simulink model "Proper"  (R2018b)
settings: Solver=VariableStepAuto  StartTime=0.0  StopTime=20.0  RelTol=1e-3
values from neighbouring files (symbols this model uses):
  g = 9.81    [ABS.m]    (also in dane.m)
  Jw = 0.01    [ABS.m]    (also in dane.m)
  K = 1000    [ABS.m]
  mv = 1200    [ABS.m]    (also in dane.m)
  roadType = 1    [ABS.m]
  rw = 0.28    [ABS.m]    (also in dane.m = 0.3)
  T = 0.01    [ABS.m]
  Tbmax = 2000    [ABS.m]
  v0 = 28    [ABS.m]
  vmin = 1.4    [ABS.m]
settings Model: Creator=Bartlomiej Mroz  LastModifiedBy=Bartlomiej Mroz

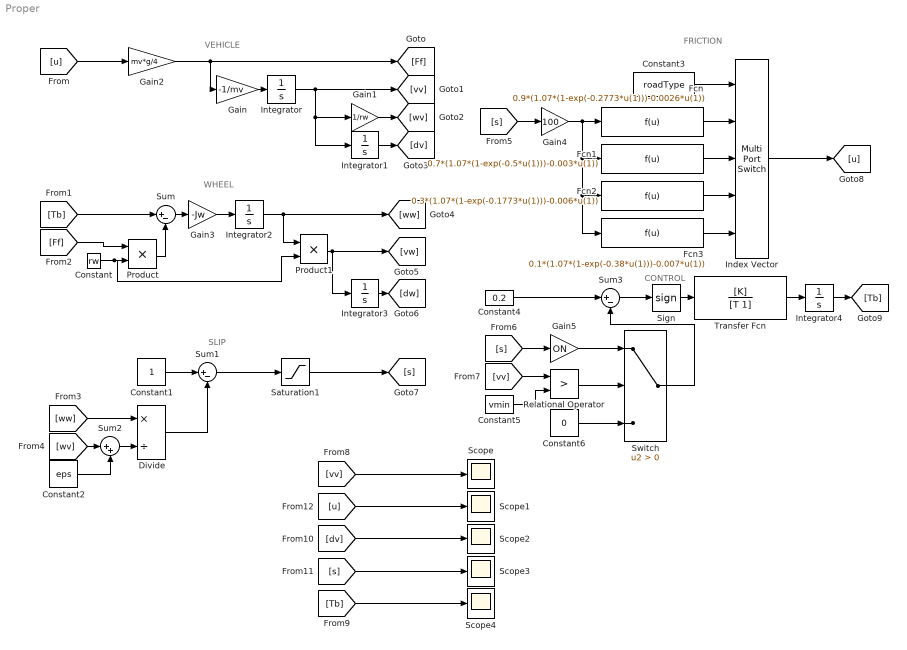
== system Proper ==
  note: CONTROL
  note: FRICTION
  note: SLIP
  note: WHEEL
  note: VEHICLE
  Constant : Constant  Value=rw
  Constant1 : Constant
  Constant2 : Constant  Value=eps
  Constant3 : Constant  Value=roadType
  Constant4 : Constant  Value=0.2
  Constant5 : Constant  Value=vmin
  Constant6 : Constant  Value=0
  Divide : Product  Inputs=*/
  Fcn : Fcn  Expr=0.9*(1.07*(1-exp(-0.2773*u(1)))-0.0026*u(1))
  Fcn1 : Fcn  Expr=0.7*(1.07*(1-exp(-0.5*u(1)))-0.003*u(1))
  Fcn2 : Fcn  Expr=0.3*(1.07*(1-exp(-0.1773*u(1)))-0.006*u(1))
  Fcn3 : Fcn  Expr=0.1*(1.07*(1-exp(-0.38*u(1)))-0.007*u(1))
  Gain : Gain  Gain=-1/mv
  Gain1 : Gain  Gain=1/rw
  Gain2 : Gain  Gain=mv*g/4
  Gain3 : Gain  Gain=-Jw
  Gain4 : Gain  Gain=100
  Gain5 : Gain  Gain=ON
  Index Vector : MultiPortSwitch  Inputs=4
  Integrator : Integrator  InitialCondition=v0  LimitOutput=on  UpperSaturationLimit=1000  LowerSaturationLimit=0
  Integrator1 : Integrator
  Integrator2 : Integrator  InitialCondition=v0/rw  LimitOutput=on  UpperSaturationLimit=1000  LowerSaturationLimit=0
  Integrator3 : Integrator
  Integrator4 : Integrator  LimitOutput=on  UpperSaturationLimit=Tbmax  LowerSaturationLimit=0
  Product : Product
  Product1 : Product
  Relational Operator : RelationalOperator  Operator=>  OutDataTypeStr=boolean  RndMeth=Simplest
  Saturation1 : Saturate  UpperLimit=1  LowerLimit=0
  Scope{,1..4} (5 alike) : Scope
  Sign : Signum
  Sum : Sum  Inputs=|+-
  Sum1 : Sum  Inputs=|+-
  Sum2 : Sum  Inputs=|++
  Sum3 : Sum  Inputs=|+-
  Switch : Switch  Criteria=u2 > Threshold
  Transfer Fcn : TransferFcn  Numerator=[K]  Denominator=[T 1]
  wires:
  [s] -> Gain4/1
  Gain4/1 -> Fcn1/1, Fcn3/1, Fcn2/1, Fcn/1
  Constant3/1 -> Index Vector/1
  Fcn/1 -> Index Vector/2
  Fcn1/1 -> Index Vector/3
  Fcn2/1 -> Index Vector/4
  Fcn3/1 -> Index Vector/5
  Constant4/1 -> Sum3/1
  [s] -> Gain5/1
  [vv] -> Relational Operator/1
  Constant5/1 -> Relational Operator/2
  Constant6/1 -> Switch/3
  Switch/1 -> Sum3/2
  [vv] -> Scope/1
  [u] -> Scope1/1
  [dv] -> Scope2/1
  [s] -> Scope3/1
  [Tb] -> Scope4/1
  Relational Operator/1 -> Switch/2
  Gain5/1 -> Switch/1
  Index Vector/1 -> [u]
  [u] -> Gain2/1
  Integrator/1 -> [vv], Integrator1/1, Gain1/1
  Gain2/1 -> [Ff], Gain/1
  Gain/1 -> Integrator/1
  Gain1/1 -> [wv]
  Integrator1/1 -> [dv]
  Product/1 -> Sum/2
  Product1/1 -> [vw], Integrator3/1
  Integrator2/1 -> [ww], Product1/1
  Gain3/1 -> Integrator2/1
  Sum/1 -> Gain3/1
  [Ff] -> Product/1
  [Tb] -> Sum/1
  Integrator3/1 -> [dw]
  Constant/1 -> Product1/2, Product/2
  Saturation1/1 -> [s]
  Sum1/1 -> Saturation1/1
  [ww] -> Divide/1
  Constant1/1 -> Sum1/1
  Divide/1 -> Sum1/2
  Sign/1 -> Transfer Fcn/1
  Transfer Fcn/1 -> Integrator4/1
  Sum3/1 -> Sign/1
  Integrator4/1 -> [Tb]
  [wv] -> Sum2/1
  Sum2/1 -> Divide/2
  Constant2/1 -> Sum2/2
